simulink model "lab2_fixed"  (R2022a)
settings: Solver=VariableStepAuto  StartTime=0.0  StopTime=10.0  RelTol=1e-3
settings Model: Creator=HP  LastModifiedBy=HP

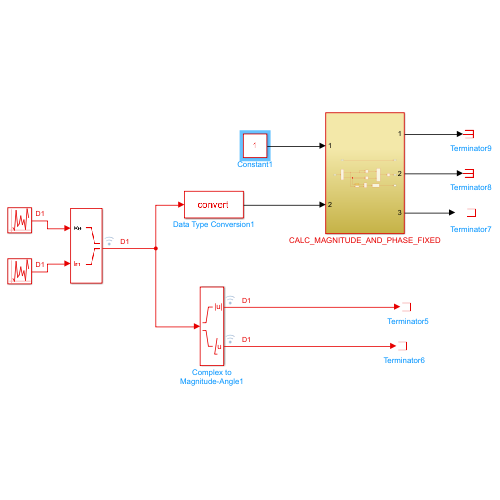
[thumbnail: Simulink's stored preview of the top-level diagram]
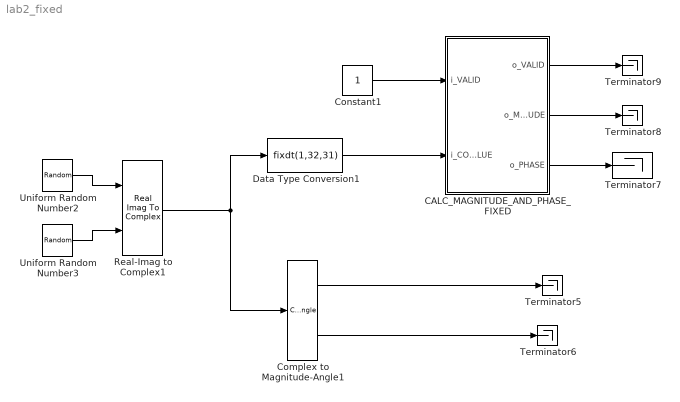
== system lab2_fixed ==
  CALC_MAGNITUDE_AND_PHASE_FIXED : Subsystem
  Complex to Magnitude-Angle1 : ComplexToMagnitudeAngle
  Constant1 : Constant  OutDataTypeStr=boolean  SampleTime=1
  Data Type Conversion1 : DataTypeConversion  OutDataTypeStr=fixdt(1,32,31)  RndMeth=Round  SaturateOnIntegerOverflow=off
  Real-Imag to Complex1 : RealImagToComplex
  Terminator{5..9} (5 alike) : Terminator
  Uniform Random Number2 : UniformRandomNumber  Minimum=0  Maximum=1.99999999953433871269  Seed=1  SampleTime=1
  Uniform Random Number3 : UniformRandomNumber  Minimum=0  Maximum=1.99999999953433871269  Seed=2  SampleTime=1
  wires:
  Uniform Random Number2/1 -> Real-Imag to Complex1/1
  Uniform Random Number3/1 -> Real-Imag to Complex1/2
  Complex to Magnitude-Angle1/1 -> Terminator5/1
  Real-Imag to Complex1/1 -> Data Type Conversion1/1, Complex to Magnitude-Angle1/1
  Complex to Magnitude-Angle1/2 -> Terminator6/1
  Constant1/1 -> CALC_MAGNITUDE_AND_PHASE_FIXED/1(i_VALID)
  Data Type Conversion1/1 -> CALC_MAGNITUDE_AND_PHASE_FIXED/2(i_COMPLEX_VALUE)
  CALC_MAGNITUDE_AND_PHASE_FIXED/3(o_PHASE) -> Terminator7/1
  CALC_MAGNITUDE_AND_PHASE_FIXED/2(o_MAGNITUDE) -> Terminator8/1
  CALC_MAGNITUDE_AND_PHASE_FIXED/1(o_VALID) -> Terminator9/1

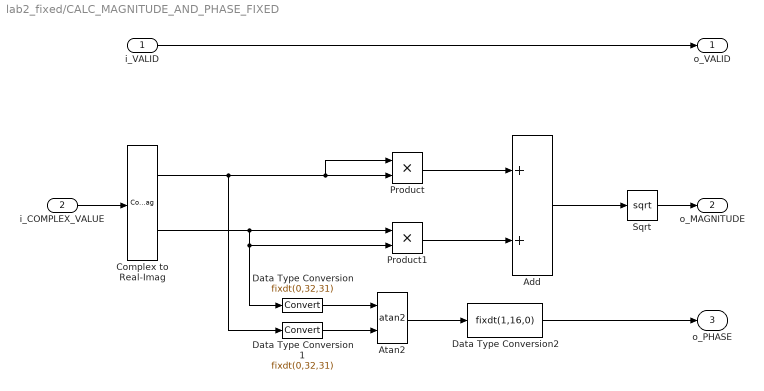
== system lab2_fixed/CALC_MAGNITUDE_AND_PHASE_FIXED ==
  i_VALID : Inport  OutDataTypeStr=boolean
  i_COMPLEX_VALUE : Inport  Port=2
  Add : Sum  OutDataTypeStr=fixdt(1,65,36)
  Atan2 : Trigonometry  Operator=atan2  ApproximationMethod=CORDIC  NumberOfIterations=20
  Complex to Real-Imag : ComplexToRealImag
  Data Type Conversion : DataTypeConversion  OutDataTypeStr=fixdt(0,32,31)  SaturateOnIntegerOverflow=off  RndMeth=Floor
  Data Type Conversion1 : DataTypeConversion  OutDataTypeStr=fixdt(0,32,31)  SaturateOnIntegerOverflow=off  RndMeth=Floor
  Data Type Conversion2 : DataTypeConversion  OutDataTypeStr=fixdt(1,16,0)  SaturateOnIntegerOverflow=off  RndMeth=Floor
  Product : Product  SaturateOnIntegerOverflow=on
  Product1 : Product  LockScale=on
  Sqrt : Sqrt  OutDataTypeStr=fixdt(1,33,31)
  o_VALID : Outport  OutDataTypeStr=boolean
  o_MAGNITUDE : Outport  Port=2
  o_PHASE : Outport  Port=3
  wires:
  Complex to Real-Imag/1 -> Data Type Conversion1/1, Product/1, Product/2
  Complex to Real-Imag/2 -> Product1/1, Product1/2, Data Type Conversion/1
  Data Type Conversion/1 -> Atan2/1
  Data Type Conversion1/1 -> Atan2/2
  Atan2/1 -> Data Type Conversion2/1
  Data Type Conversion2/1 -> o_PHASE/1
  Product1/1 -> Add/2
  Product/1 -> Add/1
  Add/1 -> Sqrt/1
  Sqrt/1 -> o_MAGNITUDE/1
  i_COMPLEX_VALUE/1 -> Complex to Real-Imag/1
  i_VALID/1 -> o_VALID/1
